simulink model "truthtable_func_test"  (R2019b)
settings: Solver=VariableStepAuto  StartTime=0.0  StopTime=10.0  RelTol=1e-3
settings Model: Creator=sasat  LastModifiedBy=sasat
settings ConfigComp: CovEnable=on  CovScope=ReferencedModels  CovIncludeTopModel=off  CovMetricSettings=dcwe  CovModelRefEnable=filtered

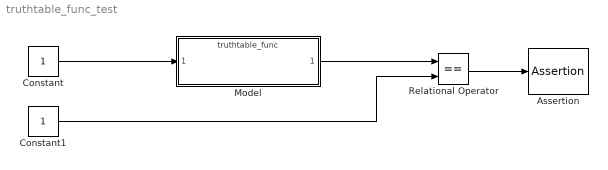
== system truthtable_func_test ==
  Assertion : Assertion
  Constant : Constant
  Constant1 : Constant
  Model : ModelReference  ModelNameDialog=truthtable_func  ModelReferenceVersion=1.6
  Relational Operator : RelationalOperator  Operator===  OutDataTypeStr=boolean  RndMeth=Simplest
  wires:
  Constant/1 -> Model/1
  Model/1 -> Relational Operator/1
  Constant1/1 -> Relational Operator/2
  Relational Operator/1 -> Assertion/1
